simulink model "lab3_s"  (R2018b)
settings: Solver=VariableStepAuto  StartTime=0.0  StopTime=t_max  MaxStep=0.1  RelTol=1e-3
values from neighbouring files (symbols this model uses):
  k = 5    [lab3.m]
  k2 = 0.33    [lab3.m]
  Lo = [1]    [lab3.m]
  Mo = [1, 3, 3, 1]    [lab3.m]
  t0 = 0    [lab3.m]
  y0 = 1    [lab3.m]
settings Model: Creator=lev  LastModifiedBy=lev

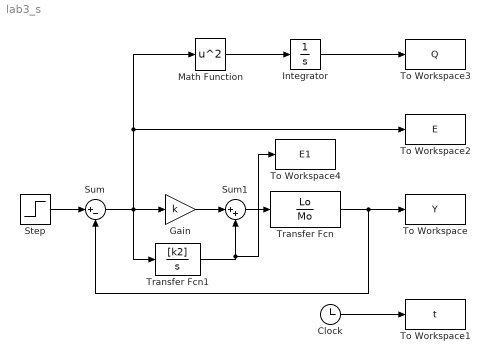
== system lab3_s ==
  Clock : Clock
  Gain : Gain  Gain=k
  Integrator : Integrator
  Math Function : Math  Operator=square  SaturateOnIntegerOverflow=on
  Step : Step  Time=t0  After=y0  SampleTime=0
  Sum : Sum  Inputs=|+-
  Sum1 : Sum  Inputs=|++
  To Workspace : ToWorkspace  VariableName=Y  SampleTime=-1
  To Workspace1 : ToWorkspace  VariableName=t  SampleTime=-1
  To Workspace2 : ToWorkspace  VariableName=E  SampleTime=-1
  To Workspace3 : ToWorkspace  VariableName=Q  SampleTime=-1
  To Workspace4 : ToWorkspace  VariableName=E1  SampleTime=-1
  Transfer Fcn : TransferFcn  Numerator=Lo  Denominator=Mo
  Transfer Fcn1 : TransferFcn  Numerator=[k2]  Denominator=[1 0]
  wires:
  Transfer Fcn/1 -> Sum/2, To Workspace/1
  Clock/1 -> To Workspace1/1
  Sum/1 -> Math Function/1, To Workspace2/1, Transfer Fcn1/1, Gain/1
  Step/1 -> Sum/1
  Sum1/1 -> Transfer Fcn/1
  Transfer Fcn1/1 -> To Workspace4/1, Sum1/2
  Gain/1 -> Sum1/1
  Math Function/1 -> Integrator/1
  Integrator/1 -> To Workspace3/1
